simulink model "SimulinkComunicacion"  (R2015b)
settings: Solver=ode45  StartTime=0.0  StopTime=10.0  RelTol=1e-3
undefined symbols (not defined in the file): serial
libraries: instrumentlib x3
settings Model: Creator=nico  LastModifiedBy=nico
settings DataIOCC: SaveFormat=Array
settings DebuggingCC: UnderspecifiedInitializationDetection=Classic  MergeDetectMultiDrivingBlocksExec=none  SolverPrmCheckMsg=warning
settings HardwareCC: ProdBitPerPointer=32  ProdLargestAtomicFloat=None  ProdIntDivRoundTo=Undefined  ProdEndianess=Unspecified  ProdWordSize=32  ProdHWDeviceType=32-bit Generic
settings GRTTargetCC: GeneratePreprocessorConditionals=Disable all
settings ConfigComp: CovModelRefEnable=Off

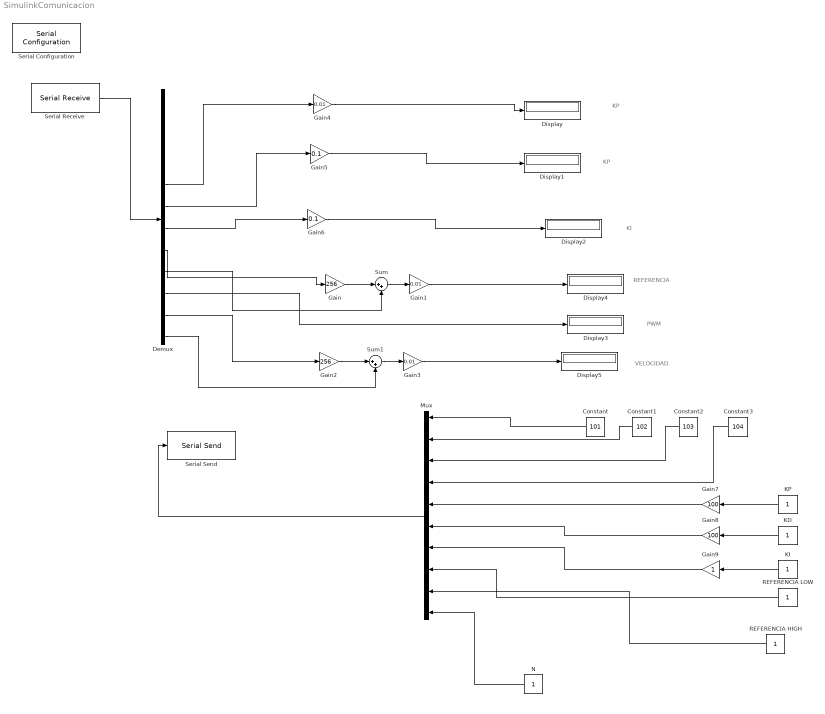
== system SimulinkComunicacion ==
  note: VELOCIDAD
  note: PWM
  note: REFERENCIA
  note: KI
  note: KP
  note: KP
  Constant : Constant  Value=101
  Constant1 : Constant  Value=102
  Constant2 : Constant  Value=103
  Constant3 : Constant  Value=104
  Demux : Demux  Outputs=12
  Display{,1..5} (6 alike) : Display
  Gain : Gain  Gain=256
  Gain1 : Gain  Gain=0.01
  Gain2 : Gain  Gain=256
  Gain3 : Gain  Gain=0.01
  Gain4 : Gain  Gain=0.01
  Gain5 : Gain  Gain=0.1
  Gain6 : Gain  Gain=0.1
  Gain7 : Gain  Gain=100
  Gain8 : Gain  Gain=100
  Gain9 : Gain
  KD : Constant
  KI : Constant
  KP : Constant
  Mux : Mux  Inputs=10
  N : Constant
  REFERENCIA HIGH : Constant
  "REFERENCIA LOW " : Constant
  Serial Configuration : instrumentlib/Serial Configuration  Priority=-200000  ComPortMenu=COM3  ComPort=COM3  ObjConstructor=serial('COM3');  BaudRate=9600  DataBits=8  Parity=none  StopBits=1  FlowControl=none  Timeout=20  ByteOrder=LittleEndian
  Serial Receive : instrumentlib/Serial Receive  ComPortMenu=COM3  ComPort=COM3  ObjConstructor=serial('COM3');  Terminator=<none>  DataSize="[12   1]"  DataType=uint8  EnableBlockingMode=on  ActionDataUnavailable=Output last received value  CustomValue=0  SampleTime=0.01
  Serial Send : instrumentlib/Serial Send  ComPortMenu=COM3  ComPort=COM3  ObjConstructor=serial('COM3');  Header=efgh  Terminator=<none>  EnableBlockingMode=on
  Sum : Sum  Inputs=|++
  Sum1 : Sum  Inputs=|++
  wires:
  Serial Receive/1 -> Demux/1
  Demux/10 -> Display3/1
  Demux/8 -> Gain/1
  Gain/1 -> Sum/1
  Demux/9 -> Sum/2
  Sum/1 -> Gain1/1
  Gain1/1 -> Display4/1
  Gain2/1 -> Sum1/1
  Sum1/1 -> Gain3/1
  Gain3/1 -> Display5/1
  Demux/11 -> Gain2/1
  Demux/12 -> Sum1/2
  Gain4/1 -> Display/1
  Demux/5 -> Gain4/1
  Gain5/1 -> Display1/1
  Demux/6 -> Gain5/1
  Gain6/1 -> Display2/1
  Demux/7 -> Gain6/1
  Constant/1 -> Mux/1
  Constant1/1 -> Mux/2
  Constant2/1 -> Mux/3
  Constant3/1 -> Mux/4
  KP/1 -> Gain7/1
  Gain7/1 -> Mux/5
  Mux/1 -> Serial Send/1
  KD/1 -> Gain8/1
  Gain8/1 -> Mux/6
  KI/1 -> Gain9/1
  Gain9/1 -> Mux/7
  "REFERENCIA LOW "/1 -> Mux/8
  N/1 -> Mux/10
  REFERENCIA HIGH/1 -> Mux/9
